simulink model "three_closedloop"  (R2023a)
settings: Solver=ode5  StartTime=0.0  StopTime=inf  FixedStep=0.001  RelTol=1e-3
undefined symbols (not defined in the file or in its folder): DiscIntNeverNeededParam, LF
libraries: simulink x10, instrumentseriallib x6, eeGeneralControl x4, sldrtlib x1
settings Model: Creator=DELL  LastModifiedBy=DELL
settings HardwareCC: ProdBitPerLong=64  ProdHWDeviceType=Intel->x86-64 (Linux 64)
settings ModelReferenceCC: EnableRefExpFcnMdlSchedulingChecks=on
settings RTWCC: Description=Simulink Desktop Real-Time  SystemTargetFile=sldrt.tlc  TemplateMakefile=sldrt.tmf  RTWCompilerOptimization=on
settings CodeAppCC: MaxIdLength=95
settings SimulinkDesktopRealTimeCC: TargetLibSuffix=_sldrt.a  TargetPreCompLibLocation=C:\Program Files\MATLAB\R2023a\toolbox\sldrt\lib\win64

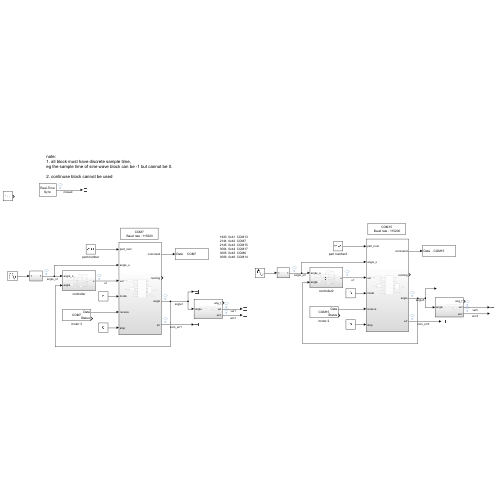
[thumbnail: Simulink's stored preview of the top-level diagram]
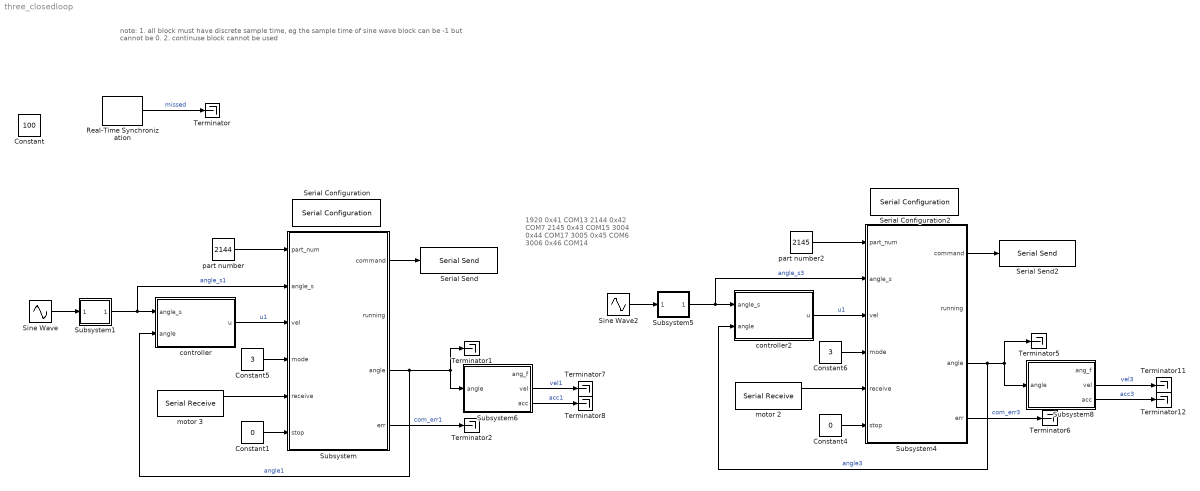
== system three_closedloop ==
  note: note:
      | 1. all block must have discrete sample time,
      | eg the sample time of sine wave block can be -1 but cannot be 0.
      |
      | 2. continuse block cannot be used
  note: 1920  0x41  COM13
      | 2144  0x42  COM7
      | 2145  0x43  COM15
      | 3004  0x44  COM17
      | 3005  0x45  COM6
      | 3006  0x46  COM14
  Constant : Constant  Value=100
  Constant1 : Constant  Value=0
  Constant4 : Constant  Value=0
  Constant5 : Constant  Value=3
  Constant6 : Constant  Value=3
  Real-Time Synchronization : sldrtlib/Real-Time Synchronization  SampleTime=0.01  MaxMissedTicks=inf  ShowMissedTicks=on  YieldWhenWaiting=off
  Serial Configuration : instrumentseriallib/Serial Configuration  Priority=-200000  PortSel=COM7  Port=COM7  ComPort=COM7  BaudRate=115200  DataBits=8  Parity=none  StopBits=1  ByteOrder=little-endian  FlowControl=none  Timeout=10  SimulateUsing=Interpreted execution  BlockInModel=on  aMode=1
  Serial Configuration2 : instrumentseriallib/Serial Configuration  Priority=-200000  PortSel=COM15  Port=COM15  ComPort=COM15  BaudRate=115200  DataBits=8  Parity=none  StopBits=1  ByteOrder=little-endian  FlowControl=none  Timeout=10  SimulateUsing=Interpreted execution  BlockInModel=on  aMode=1
  Serial Send : instrumentseriallib/Serial Send  Priority=1  PortSel=COM7  Port=COM7  ComPort=COM7  Header=[]  Terminator=<none>  CustomTerminator=[]  EnableBlockingMode=off  SimulateUsing=Interpreted execution  BlockInModel=on  aMode=1
  Serial Send2 : instrumentseriallib/Serial Send  Priority=1  PortSel=COM15  Port=COM15  ComPort=COM15  Header=[]  Terminator=<none>  CustomTerminator=[]  EnableBlockingMode=off  SimulateUsing=Interpreted execution  BlockInModel=on  aMode=1
  Sine Wave : Sin  Amplitude=15  Phase=pi/4
  Sine Wave2 : Sin  Amplitude=15
  Subsystem : Subsystem
  Subsystem1 : Subsystem
  Subsystem4 : Subsystem
  Subsystem5 : Subsystem
  Subsystem6 : Subsystem
  Subsystem8 : Subsystem
  Terminator{,1..2,5..8,11..12} (9 alike) : Terminator
  controller : Subsystem
  controller2 : Subsystem
  motor 2 : instrumentseriallib/Serial Receive  Priority=1  PortSel=COM15  Port=COM15  ComPort=COM15  DataType=uint8  SaveDataType=uint8  ToggleHeader=off  Header=[]  ToggleTerminator=on  Terminator=LF ('\n')  CustomTerminator=[]  InputFormat=Column major  ToggleDataSize=on  DataSize=[1 7]  EnableBlockingMode=off  ActionDataUnavailable=Output last received value  ActionWhenDataUnavailable=Output last received value  CustomValue=0  SampleTime=0.005  SimulateUsing=Interpreted execution  BlockInModel=on  aMode=1
  motor 3 : instrumentseriallib/Serial Receive  Priority=1  PortSel=COM7  Port=COM7  ComPort=COM7  DataType=uint8  SaveDataType=uint8  ToggleHeader=off  Header=[]  ToggleTerminator=on  Terminator=LF ('\n')  CustomTerminator=[]  InputFormat=Column major  ToggleDataSize=on  DataSize=[1 7]  EnableBlockingMode=off  ActionDataUnavailable=Output last received value  ActionWhenDataUnavailable=Output last received value  CustomValue=0  SampleTime=0.005  SimulateUsing=Interpreted execution  BlockInModel=on  aMode=1
  part number : Constant  Value=2144
  part number2 : Constant  Value=2145
  wires:
  Subsystem1/1(Out1) -> Subsystem/2(angle_s), controller/1(angle_s)  "angle_s1"
  Subsystem/3(angle) -> Subsystem6/1(angle), Terminator1/1, controller/2(angle)  "angle1"
  part number/1 -> Subsystem/1(part_num)
  Constant5/1 -> Subsystem/4(mode)
  motor 3/1 -> Subsystem/5(receive)
  Subsystem/1(command) -> Serial Send/1
  Subsystem/4(err) -> Terminator2/1  "com_err1"
  controller/1(u) -> Subsystem/3(vel)  "u1"
  Sine Wave/1 -> Subsystem1/1(In1)
  Real-Time Synchronization/1 -> Terminator/1  "missed"
  Constant1/1 -> Subsystem/6(stop)
  Constant6/1 -> Subsystem4/4(mode)
  motor 2/1 -> Subsystem4/5(receive)
  part number2/1 -> Subsystem4/1(part_num)
  controller2/1(u) -> Subsystem4/3(vel)  "u1"
  Subsystem4/1(command) -> Serial Send2/1
  Subsystem4/3(angle) -> Subsystem8/1(angle), Terminator5/1, controller2/2(angle)  "angle3"
  Constant4/1 -> Subsystem4/6(stop)
  Subsystem4/4(err) -> Terminator6/1  "com_err3"
  Subsystem5/1(Out1) -> Subsystem4/2(angle_s), controller2/1(angle_s)  "angle_s3"
  Sine Wave2/1 -> Subsystem5/1(In1)
  Subsystem6/2(vel) -> Terminator7/1  "vel1"
  Subsystem6/3(acc) -> Terminator8/1  "acc1"
  Subsystem8/2(vel) -> Terminator11/1  "vel3"
  Subsystem8/3(acc) -> Terminator12/1  "acc3"

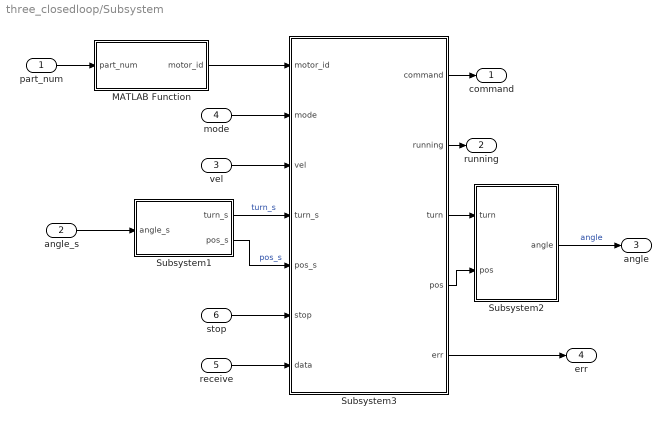
== system three_closedloop/Subsystem ==
  part_num : Inport
  angle_s : Inport  Port=2
  vel : Inport  Port=3
  mode : Inport  Port=4
  receive : Inport  Port=5
  stop : Inport  Port=6
  MATLAB Function : MATLAB Function  TreatAsAtomicUnit=on
  Subsystem1 : Subsystem
  Subsystem2 : Subsystem
  Subsystem3 : Subsystem
  command : Outport
  running : Outport  Port=2
  angle : Outport  Port=3
  err : Outport  Port=4
  wires:
  Subsystem3/4(pos) -> Subsystem2/2(pos)
  Subsystem1/1(turn_s) -> Subsystem3/4(turn_s)  "turn_s"
  Subsystem1/2(pos_s) -> Subsystem3/5(pos_s)  "pos_s"
  MATLAB Function/1(motor_id) -> Subsystem3/1(motor_id)
  part_num/1 -> MATLAB Function/1(part_num)
  Subsystem3/3(turn) -> Subsystem2/1(turn)
  Subsystem2/1(angle) -> angle/1  "angle"
  angle_s/1 -> Subsystem1/1(angle_s)
  Subsystem3/5(err) -> err/1
  Subsystem3/2(running) -> running/1
  receive/1 -> Subsystem3/7(data)
  vel/1 -> Subsystem3/3(vel)
  Subsystem3/1(command) -> command/1
  mode/1 -> Subsystem3/2(mode)
  stop/1 -> Subsystem3/6(stop)

== system three_closedloop/Subsystem1 ==
  In1 : Inport
  Out1 : Outport
  wires:
  In1/1 -> Out1/1

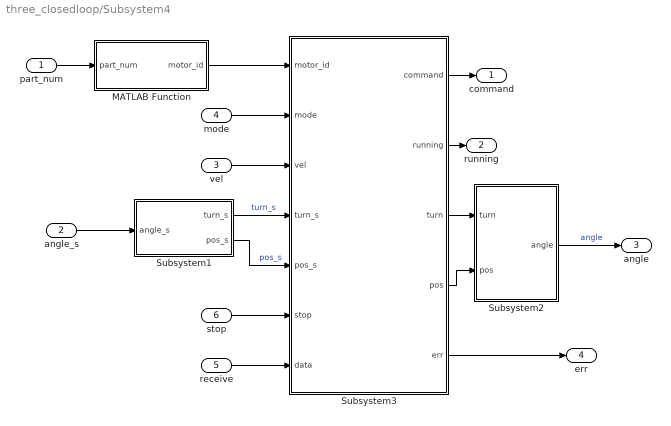
== system three_closedloop/Subsystem4 ==
  part_num : Inport
  angle_s : Inport  Port=2
  vel : Inport  Port=3
  mode : Inport  Port=4
  receive : Inport  Port=5
  stop : Inport  Port=6
  MATLAB Function : MATLAB Function  TreatAsAtomicUnit=on
  Subsystem1 : Subsystem
  Subsystem2 : Subsystem
  Subsystem3 : Subsystem
  command : Outport
  running : Outport  Port=2
  angle : Outport  Port=3
  err : Outport  Port=4
  wires:
  Subsystem3/4(pos) -> Subsystem2/2(pos)
  Subsystem1/1(turn_s) -> Subsystem3/4(turn_s)  "turn_s"
  Subsystem1/2(pos_s) -> Subsystem3/5(pos_s)  "pos_s"
  MATLAB Function/1(motor_id) -> Subsystem3/1(motor_id)
  part_num/1 -> MATLAB Function/1(part_num)
  Subsystem3/3(turn) -> Subsystem2/1(turn)
  Subsystem2/1(angle) -> angle/1  "angle"
  angle_s/1 -> Subsystem1/1(angle_s)
  Subsystem3/5(err) -> err/1
  Subsystem3/2(running) -> running/1
  receive/1 -> Subsystem3/7(data)
  vel/1 -> Subsystem3/3(vel)
  Subsystem3/1(command) -> command/1
  mode/1 -> Subsystem3/2(mode)
  stop/1 -> Subsystem3/6(stop)

== system three_closedloop/Subsystem5 ==
  In1 : Inport
  Out1 : Outport
  wires:
  In1/1 -> Out1/1

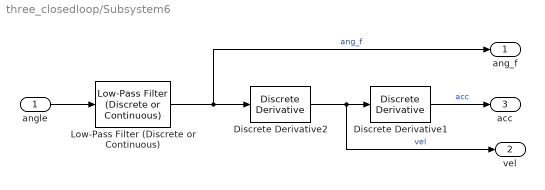
== system three_closedloop/Subsystem6 ==
  angle : Inport
  Discrete Derivative1 : simulink/Discrete/Discrete Derivative  gainval=1.0  ICPrevScaledInput=0.0  OutMin=[]  OutMax=[]  OutDataType=fixdt(1, 16)  OutScaling=2^-10  DoSatur=off
  Discrete Derivative2 : simulink/Discrete/Discrete Derivative  gainval=1.0  ICPrevScaledInput=0.0  OutMin=[]  OutMax=[]  OutDataType=fixdt(1, 16)  OutScaling=2^-10  DoSatur=off
  Low-Pass Filter (Discrete or Continuous) : eeGeneralControl/Low-Pass Filter (Discrete or Continuous)  K=1  T=0.1  B=inf  A=-inf  init_option=Inherited from block input  x0=0  Ts=-1
  ang_f : Outport
  vel : Outport  Port=2
  acc : Outport  Port=3
  wires:
  Discrete Derivative2/1 -> vel/1, Discrete Derivative1/1  "vel"
  Low-Pass Filter (Discrete or Continuous)/1 -> ang_f/1, Discrete Derivative2/1  "ang_f"
  angle/1 -> Low-Pass Filter (Discrete or Continuous)/1
  Discrete Derivative1/1 -> acc/1  "acc"

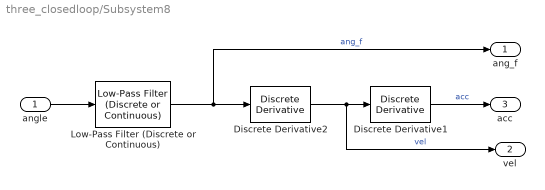
== system three_closedloop/Subsystem8 ==
  angle : Inport
  Discrete Derivative1 : simulink/Discrete/Discrete Derivative  gainval=1.0  ICPrevScaledInput=0.0  OutMin=[]  OutMax=[]  OutDataType=fixdt(1, 16)  OutScaling=2^-10  DoSatur=off
  Discrete Derivative2 : simulink/Discrete/Discrete Derivative  gainval=1.0  ICPrevScaledInput=0.0  OutMin=[]  OutMax=[]  OutDataType=fixdt(1, 16)  OutScaling=2^-10  DoSatur=off
  Low-Pass Filter (Discrete or Continuous) : eeGeneralControl/Low-Pass Filter (Discrete or Continuous)  K=1  T=0.1  B=inf  A=-inf  init_option=Inherited from block input  x0=0  Ts=-1
  ang_f : Outport
  vel : Outport  Port=2
  acc : Outport  Port=3
  wires:
  Discrete Derivative2/1 -> vel/1, Discrete Derivative1/1  "vel"
  Low-Pass Filter (Discrete or Continuous)/1 -> ang_f/1, Discrete Derivative2/1  "ang_f"
  angle/1 -> Low-Pass Filter (Discrete or Continuous)/1
  Discrete Derivative1/1 -> acc/1  "acc"

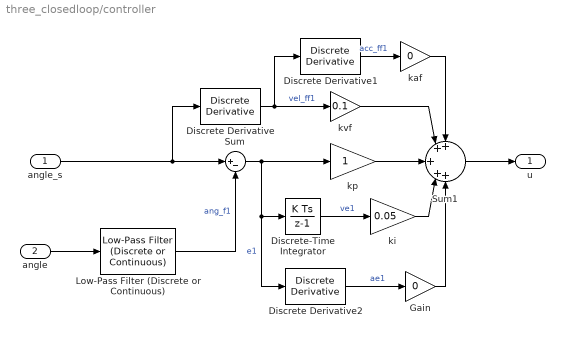
== system three_closedloop/controller ==
  angle_s : Inport
  angle : Inport  Port=2
  Discrete Derivative : simulink/Discrete/Discrete Derivative  gainval=1.0  ICPrevScaledInput=0.0  OutMin=[]  OutMax=[]  OutDataType=fixdt(1, 16)  OutScaling=2^-10  DoSatur=off
  Discrete Derivative1 : simulink/Discrete/Discrete Derivative  gainval=1.0  ICPrevScaledInput=0.0  OutMin=[]  OutMax=[]  OutDataType=fixdt(1, 16)  OutScaling=2^-10  DoSatur=off
  Discrete Derivative2 : simulink/Discrete/Discrete Derivative  gainval=1.0  ICPrevScaledInput=0.0  OutMin=[]  OutMax=[]  OutDataType=fixdt(1, 16)  OutScaling=2^-10  DoSatur=off
  Discrete-Time Integrator : DiscreteIntegrator  SampleTime=-1  ICPrevOutput=DiscIntNeverNeededParam  ICPrevScaledInput=DiscIntNeverNeededParam
  Gain : Gain  Gain=0
  Low-Pass Filter (Discrete or Continuous) : eeGeneralControl/Low-Pass Filter (Discrete or Continuous)  K=1  T=0.1  B=inf  A=-inf  init_option=Inherited from block input  x0=0  Ts=-1
  Sum : Sum  Inputs=|+-
  Sum1 : Sum  Inputs=++|+|++
  kaf : Gain  Gain=0
  ki : Gain  Gain=0.05
  kp : Gain
  kvf : Gain  Gain=0.1
  u : Outport
  wires:
  Sum1/1 -> u/1
  Sum/1 -> Discrete Derivative2/1, Discrete-Time Integrator/1, kp/1  "e1"
  Discrete Derivative1/1 -> kaf/1  "acc_ff1"
  Discrete Derivative/1 -> kvf/1, Discrete Derivative1/1  "vel_ff1"
  kaf/1 -> Sum1/1
  kvf/1 -> Sum1/2
  kp/1 -> Sum1/3
  angle_s/1 -> Discrete Derivative/1, Sum/1
  angle/1 -> Low-Pass Filter (Discrete or Continuous)/1
  Low-Pass Filter (Discrete or Continuous)/1 -> Sum/2  "ang_f1"
  Discrete-Time Integrator/1 -> ki/1  "ve1"
  ki/1 -> Sum1/4
  Discrete Derivative2/1 -> Gain/1  "ae1"
  Gain/1 -> Sum1/5

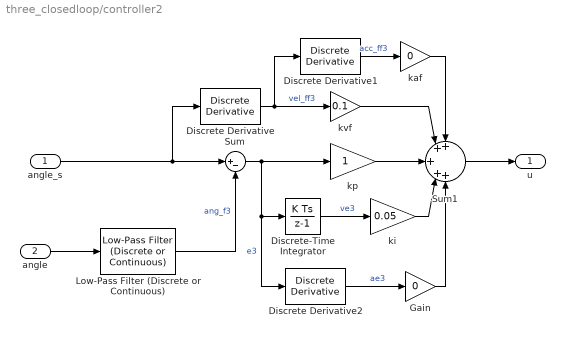
== system three_closedloop/controller2 ==
  angle_s : Inport
  angle : Inport  Port=2
  Discrete Derivative : simulink/Discrete/Discrete Derivative  gainval=1.0  ICPrevScaledInput=0.0  OutMin=[]  OutMax=[]  OutDataType=fixdt(1, 16)  OutScaling=2^-10  DoSatur=off
  Discrete Derivative1 : simulink/Discrete/Discrete Derivative  gainval=1.0  ICPrevScaledInput=0.0  OutMin=[]  OutMax=[]  OutDataType=fixdt(1, 16)  OutScaling=2^-10  DoSatur=off
  Discrete Derivative2 : simulink/Discrete/Discrete Derivative  gainval=1.0  ICPrevScaledInput=0.0  OutMin=[]  OutMax=[]  OutDataType=fixdt(1, 16)  OutScaling=2^-10  DoSatur=off
  Discrete-Time Integrator : DiscreteIntegrator  SampleTime=-1  ICPrevOutput=DiscIntNeverNeededParam  ICPrevScaledInput=DiscIntNeverNeededParam
  Gain : Gain  Gain=0
  Low-Pass Filter (Discrete or Continuous) : eeGeneralControl/Low-Pass Filter (Discrete or Continuous)  K=1  T=0.1  B=inf  A=-inf  init_option=Inherited from block input  x0=0  Ts=-1
  Sum : Sum  Inputs=|+-
  Sum1 : Sum  Inputs=++|+|++
  kaf : Gain  Gain=0
  ki : Gain  Gain=0.05
  kp : Gain
  kvf : Gain  Gain=0.1
  u : Outport
  wires:
  Sum1/1 -> u/1
  Sum/1 -> Discrete Derivative2/1, Discrete-Time Integrator/1, kp/1  "e3"
  Discrete Derivative1/1 -> kaf/1  "acc_ff3"
  Discrete Derivative/1 -> kvf/1, Discrete Derivative1/1  "vel_ff3"
  kaf/1 -> Sum1/1
  kvf/1 -> Sum1/2
  kp/1 -> Sum1/3
  angle_s/1 -> Discrete Derivative/1, Sum/1
  angle/1 -> Low-Pass Filter (Discrete or Continuous)/1
  Low-Pass Filter (Discrete or Continuous)/1 -> Sum/2  "ang_f3"
  Discrete-Time Integrator/1 -> ki/1  "ve3"
  ki/1 -> Sum1/4
  Discrete Derivative2/1 -> Gain/1  "ae3"
  Gain/1 -> Sum1/5

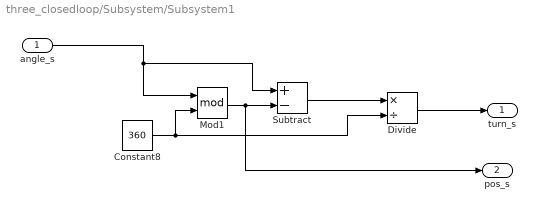
== system three_closedloop/Subsystem/Subsystem1 ==
  angle_s : Inport
  Constant8 : Constant  Value=360
  Divide : Product  Inputs=*/
  Mod1 : Math  Operator=mod
  Subtract : Sum  Inputs=+-
  turn_s : Outport
  pos_s : Outport  Port=2
  wires:
  Constant8/1 -> Divide/2, Mod1/2
  angle_s/1 -> Subtract/1, Mod1/1
  Mod1/1 -> pos_s/1, Subtract/2
  Subtract/1 -> Divide/1
  Divide/1 -> turn_s/1

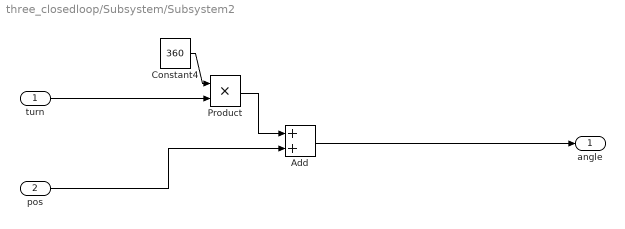
== system three_closedloop/Subsystem/Subsystem2 ==
  turn : Inport
  pos : Inport  Port=2
  Add : Sum
  Constant4 : Constant  Value=360
  Product : Product
  angle : Outport
  wires:
  turn/1 -> Product/2
  Constant4/1 -> Product/1
  Product/1 -> Add/1
  Add/1 -> angle/1
  pos/1 -> Add/2

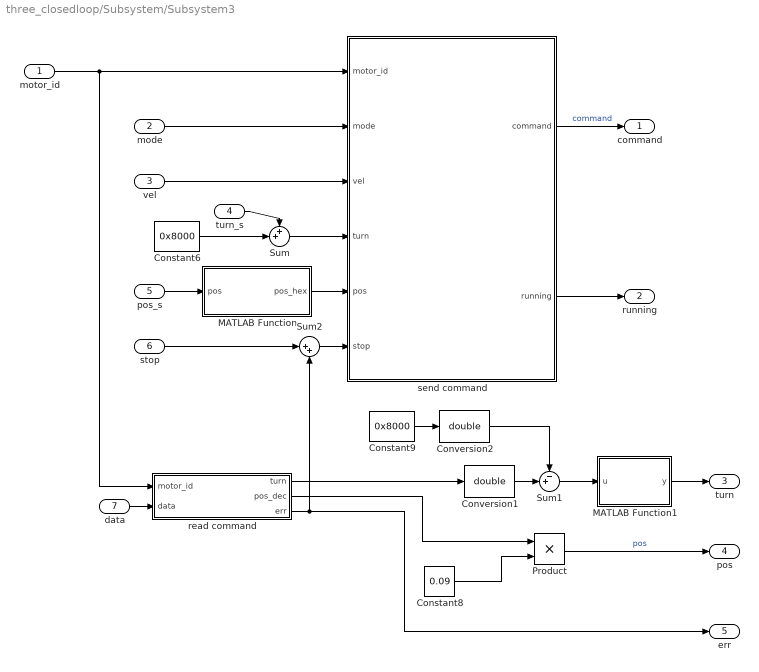
== system three_closedloop/Subsystem/Subsystem3 ==
  motor_id : Inport
  mode : Inport  Port=2
  vel : Inport  Port=3
  turn_s : Inport  Port=4
  pos_s : Inport  Port=5
  stop : Inport  Port=6
  data : Inport  Port=7
  Constant6 : Constant  Value=0x8000
  Constant8 : Constant  Value=0.09
  Constant9 : Constant  Value=0x8000
  Conversion1 : DataTypeConversion  OutDataTypeStr=double  SaturateOnIntegerOverflow=off  RndMeth=Floor
  Conversion2 : DataTypeConversion  OutDataTypeStr=double  SaturateOnIntegerOverflow=off  RndMeth=Floor
  MATLAB Function : MATLAB Function  TreatAsAtomicUnit=on
  MATLAB Function1 : MATLAB Function  TreatAsAtomicUnit=on
  Product : Product
  Sum : Sum  Inputs=++|
  Sum1 : Sum  Inputs=-+|
  Sum2 : Sum  Inputs=|++
  read command : MATLAB Function  TreatAsAtomicUnit=on
  send command : MATLAB Function  TreatAsAtomicUnit=on
  command : Outport
  running : Outport  Port=2
  turn : Outport  Port=3
  pos : Outport  Port=4
  err : Outport  Port=5
  wires:
  Constant6/1 -> Sum/2
  send command/2(running) -> running/1
  MATLAB Function/1(pos_hex) -> send command/5(pos)
  vel/1 -> send command/3(vel)
  read command/2(pos_dec) -> Product/1
  Sum/1 -> send command/4(turn)
  Constant8/1 -> Product/2
  Product/1 -> pos/1  "pos"
  data/1 -> read command/2(data)
  motor_id/1 -> read command/1(motor_id), send command/1(motor_id)
  send command/1(command) -> command/1  "command"
  pos_s/1 -> MATLAB Function/1(pos)
  mode/1 -> send command/2(mode)
  turn_s/1 -> Sum/1
  read command/1(turn) -> Conversion1/1
  Conversion1/1 -> Sum1/2
  Constant9/1 -> Conversion2/1
  Conversion2/1 -> Sum1/1
  Sum1/1 -> MATLAB Function1/1(u)
  MATLAB Function1/1(y) -> turn/1
  read command/3(err) -> err/1, Sum2/2
  stop/1 -> Sum2/1
  Sum2/1 -> send command/6(stop)

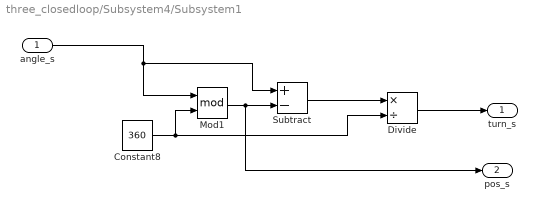
== system three_closedloop/Subsystem4/Subsystem1 ==
  angle_s : Inport
  Constant8 : Constant  Value=360
  Divide : Product  Inputs=*/
  Mod1 : Math  Operator=mod
  Subtract : Sum  Inputs=+-
  turn_s : Outport
  pos_s : Outport  Port=2
  wires:
  Constant8/1 -> Divide/2, Mod1/2
  angle_s/1 -> Subtract/1, Mod1/1
  Mod1/1 -> pos_s/1, Subtract/2
  Subtract/1 -> Divide/1
  Divide/1 -> turn_s/1

== system three_closedloop/Subsystem4/Subsystem2 ==
  turn : Inport
  pos : Inport  Port=2
  Add : Sum
  Constant4 : Constant  Value=360
  Product : Product
  angle : Outport
  wires:
  turn/1 -> Product/2
  Constant4/1 -> Product/1
  Product/1 -> Add/1
  Add/1 -> angle/1
  pos/1 -> Add/2

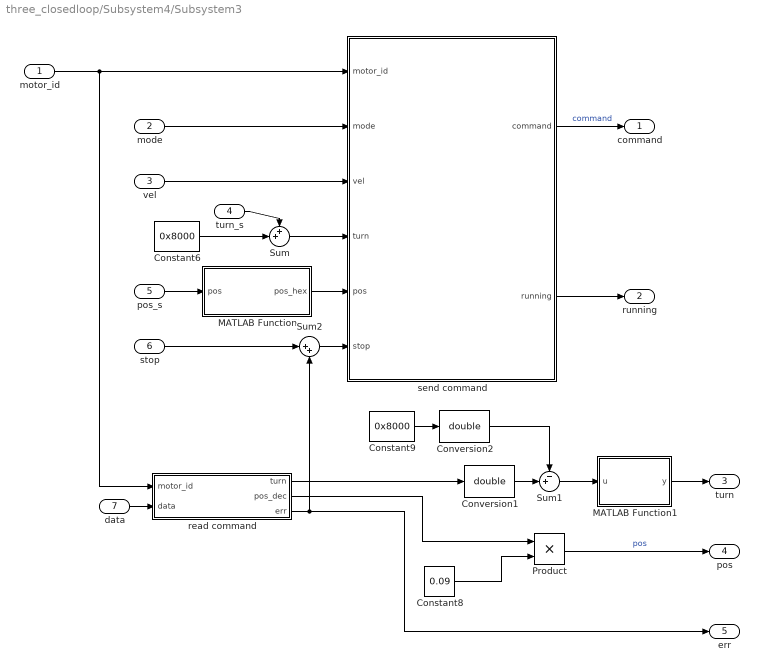
== system three_closedloop/Subsystem4/Subsystem3 ==
  motor_id : Inport
  mode : Inport  Port=2
  vel : Inport  Port=3
  turn_s : Inport  Port=4
  pos_s : Inport  Port=5
  stop : Inport  Port=6
  data : Inport  Port=7
  Constant6 : Constant  Value=0x8000
  Constant8 : Constant  Value=0.09
  Constant9 : Constant  Value=0x8000
  Conversion1 : DataTypeConversion  OutDataTypeStr=double  SaturateOnIntegerOverflow=off  RndMeth=Floor
  Conversion2 : DataTypeConversion  OutDataTypeStr=double  SaturateOnIntegerOverflow=off  RndMeth=Floor
  MATLAB Function : MATLAB Function  TreatAsAtomicUnit=on
  MATLAB Function1 : MATLAB Function  TreatAsAtomicUnit=on
  Product : Product
  Sum : Sum  Inputs=++|
  Sum1 : Sum  Inputs=-+|
  Sum2 : Sum  Inputs=|++
  read command : MATLAB Function  TreatAsAtomicUnit=on
  send command : MATLAB Function  TreatAsAtomicUnit=on
  command : Outport
  running : Outport  Port=2
  turn : Outport  Port=3
  pos : Outport  Port=4
  err : Outport  Port=5
  wires:
  Constant6/1 -> Sum/2
  send command/2(running) -> running/1
  MATLAB Function/1(pos_hex) -> send command/5(pos)
  vel/1 -> send command/3(vel)
  read command/2(pos_dec) -> Product/1
  Sum/1 -> send command/4(turn)
  Constant8/1 -> Product/2
  Product/1 -> pos/1  "pos"
  data/1 -> read command/2(data)
  motor_id/1 -> read command/1(motor_id), send command/1(motor_id)
  send command/1(command) -> command/1  "command"
  pos_s/1 -> MATLAB Function/1(pos)
  mode/1 -> send command/2(mode)
  turn_s/1 -> Sum/1
  read command/1(turn) -> Conversion1/1
  Conversion1/1 -> Sum1/2
  Constant9/1 -> Conversion2/1
  Conversion2/1 -> Sum1/1
  Sum1/1 -> MATLAB Function1/1(u)
  MATLAB Function1/1(y) -> turn/1
  read command/3(err) -> err/1, Sum2/2
  stop/1 -> Sum2/1
  Sum2/1 -> send command/6(stop)

== matlab function three_closedloop/Subsystem/MATLAB Function ==
  data: part_num input; motor_id output
function motor_id = motor_id(part_num)
%#codegen
    motor_id=0x40;
    switch part_num
        case 1920
            motor_id=0x41;
        case 2144
            motor_id=0x42;
        case 2145
            motor_id=0x43;
        case 3004
            motor_id = 0x44;
        case 3005
            motor_id = 0x45;
        case 3006
            motor_id = 0x46;
        otherwise
            motor_id = 0x40;
    end
end

== matlab function three_closedloop/Subsystem/Subsystem3/MATLAB Function ==
  data: pos input; pos_hex output
function pos_hex = fcn(pos)
pos = pos/0.09;
pos_hex = 0x0000;
mult = 1;
while pos>0
    digit = mod(pos,10);
    pos = pos - digit;
    pos = pos/10;
    pos_hex = pos_hex + uint16(mult*digit);
    mult = mult*16;
end

== matlab function three_closedloop/Subsystem/Subsystem3/MATLAB Function1 ==
  data: u input; y output
function y = adjust_init(u)
if(u<=-32767)
    y=0;
else
    y = u;
end

== matlab function three_closedloop/Subsystem/Subsystem3/read command ==
  data: motor_id input; data input; turn output; pos_dec output; err output
function [turn,pos_dec,err] = fcn(motor_id, data)
err=0;
turn=0x8000;
pos_dec=0x0000;
if data(1)~=motor_id
    err=1;
    return
end
if data(2)~=0x54
    err=2;
    return
end
turn = uint16(data(3))*0x100 + uint16(data(4));
pos = uint16(data(5))*0x100 + uint16(data(6));
pos_dec = 0x0000;
mult = 1;
while pos>0
    p1 = mod(pos,0x0010);
    pos = pos - p1;
    pos = pos/0x0010;
    pos_dec = pos_dec + p1*mult;
    mult = mult*10;
end

== matlab function three_closedloop/Subsystem/Subsystem3/send command ==
  data: motor_id input; mode input; vel input; command output; turn input; running output; pos input; stop input
function [command ,running]= fcn(motor_id, mode, vel,turn,pos,stop)
    command = uint8(zeros(1,16));
    command(9:16) = [motor_id 0x51 0 0 0 0 0 0x0A];

    command(8) = 0x0A;
    command(1) = motor_id;
    running = 1;
    % force stop
    if  stop == 1
        command(2) = 0x53;       
        running = 0;
        return        
    end

    % set mode
    switch mode
        % continues velocity loop
        case 1
            if vel>0
                command(2) = 0x44;
            elseif vel<0
                command(2)=0x55;   
            else
                command(2) = 0x53;
                running = 0;   
            end
            command(7) = abs(vel);
        % impulse velocity loop
        case 2
            if vel>0
                command(2) = 0x46;
            elseif vel<0
                command(2)=0x56;  
            else
                command(2) = 0x53;
                running = 0;                   
            end
            command(7) = abs(vel);
        % coontinue position loop
        case 3
            command(2) = 2;
            command(3) = uint8((turn-mod(turn,0x100))/0x100);
            command(4) = uint8(mod(turn,0x100));
            command(5) = uint8((pos-mod(pos,0x100))/0x100);
            command(6) = uint8(mod(pos,0x100));            
            command(7) = abs(vel);
        % impulse position loop
        case 4
            command(2) = 3;
            command(3) = uint8((turn-mod(turn,0x100))/0x100);
            command(4) = uint8(mod(turn,0x100));
            command(5) = uint8((pos-mod(pos,0x100))/0x100);
            command(6) = uint8(mod(pos,0x100));                
            command(7) = abs(vel);
        case 5
            command(2) = 0x52;
        otherwise
            command(2) = 0x53;       
            running = 0;
    end
end

== matlab function three_closedloop/Subsystem4/MATLAB Function ==
  data: part_num input; motor_id output
function motor_id = motor_id(part_num)
%#codegen
    motor_id=0x40;
    switch part_num
        case 1920
            motor_id=0x41;
        case 2144
            motor_id=0x42;
        case 2145
            motor_id=0x43;
        case 3004
            motor_id = 0x44;
        case 3005
            motor_id = 0x45;
        case 3006
            motor_id = 0x46;
        otherwise
            motor_id = 0x40;
    end
end

== matlab function three_closedloop/Subsystem4/Subsystem3/MATLAB Function ==
  data: pos input; pos_hex output
function pos_hex = fcn(pos)
pos = pos/0.09;
pos_hex = 0x0000;
mult = 1;
while pos>0
    digit = mod(pos,10);
    pos = pos - digit;
    pos = pos/10;
    pos_hex = pos_hex + uint16(mult*digit);
    mult = mult*16;
end

== matlab function three_closedloop/Subsystem4/Subsystem3/MATLAB Function1 ==
  data: u input; y output
function y = adjust_init(u)
if(u<=-32767)
    y=0;
else
    y = u;
end

== matlab function three_closedloop/Subsystem4/Subsystem3/read command ==
  data: motor_id input; data input; turn output; pos_dec output; err output
function [turn,pos_dec,err] = fcn(motor_id, data)
err=0;
turn=0x8000;
pos_dec=0x0000;
if data(1)~=motor_id
    err=1;
    return
end
if data(2)~=0x54
    err=2;
    return
end
turn = uint16(data(3))*0x100 + uint16(data(4));
pos = uint16(data(5))*0x100 + uint16(data(6));
pos_dec = 0x0000;
mult = 1;
while pos>0
    p1 = mod(pos,0x0010);
    pos = pos - p1;
    pos = pos/0x0010;
    pos_dec = pos_dec + p1*mult;
    mult = mult*10;
end

== matlab function three_closedloop/Subsystem4/Subsystem3/send command ==
  data: motor_id input; mode input; vel input; command output; turn input; running output; pos input; stop input
function [command ,running]= fcn(motor_id, mode, vel,turn,pos,stop)
    command = uint8(zeros(1,16));
    command(9:16) = [motor_id 0x51 0 0 0 0 0 0x0A];

    command(8) = 0x0A;
    command(1) = motor_id;
    running = 1;
    % force stop
    if  stop == 1
        command(2) = 0x53;       
        running = 0;
        return        
    end

    % set mode
    switch mode
        % continues velocity loop
        case 1
            if vel>0
                command(2) = 0x44;
            elseif vel<0
                command(2)=0x55;   
            else
                command(2) = 0x53;
                running = 0;   
            end
            command(7) = abs(vel);
        % impulse velocity loop
        case 2
            if vel>0
                command(2) = 0x46;
            elseif vel<0
                command(2)=0x56;  
            else
                command(2) = 0x53;
                running = 0;                   
            end
            command(7) = abs(vel);
        % coontinue position loop
        case 3
            command(2) = 2;
            command(3) = uint8((turn-mod(turn,0x100))/0x100);
            command(4) = uint8(mod(turn,0x100));
            command(5) = uint8((pos-mod(pos,0x100))/0x100);
            command(6) = uint8(mod(pos,0x100));            
            command(7) = abs(vel);
        % impulse position loop
        case 4
            command(2) = 3;
            command(3) = uint8((turn-mod(turn,0x100))/0x100);
            command(4) = uint8(mod(turn,0x100));
            command(5) = uint8((pos-mod(pos,0x100))/0x100);
            command(6) = uint8(mod(pos,0x100));                
            command(7) = abs(vel);
        case 5
            command(2) = 0x52;
        otherwise
            command(2) = 0x53;       
            running = 0;
    end
end
